simulink library "Feuchtesimulation_Lib"  (R2018b)
settings: Solver=VariableStepAuto  StartTime=0.0  StopTime=10.0  RelTol=1e-3
undefined symbols (not defined in the file or in its folder): A_Kat0, A_Mantel_Kat0, Ads_AusnutzungsFaktor, adsorptionsenthalpie, AIR_mw, beladungskennfeld, c_edelstahl, c_Isomatte, deltaH_verd, DiscIntNeverNeededParam, H2O_mw, Kat0_Anzahl_Zonen, Kond_AusnutzungsFaktor, Kond_KL_Faktor_, KondVerd_KLKF_mf_StSt_kgps, l_Kat0, m_Canning_Kat0, m_h2o_kat0_ads, m_h2o_kat0_kond, m_Isolierung_Kat0, m_zeolith_kat0_zone, m_zKat0, Mat_Kat0, mGas_imRohrabschnitt_kg, mZeo_UnterDerZeo0angenommenWird, p_dsat, R_sLuft, rate_k_verd, Rohr1, RTh_Brick_Iso_Kat0, RTh_Iso_Canning_Kat0, Sensor0, SensorIn, switch_TInit_Tstart_bei_true_sonst_TInitAusMessung, T_start, Tk0_1, ts, Verd_KF_Dampfdruck_StSt, Verd_KL_Faktor, waermekapazitaet_luft, waermekapazitaet_wasser_fluessig, waermekapazitaet_wasser_gasfoermig, WuezRohr_Dynamikfaktor
libraries: simulink x5, $bdroot x3
(part 1 of 2)
settings Model: Creator=QXS2633  LastModifiedBy=qt28407

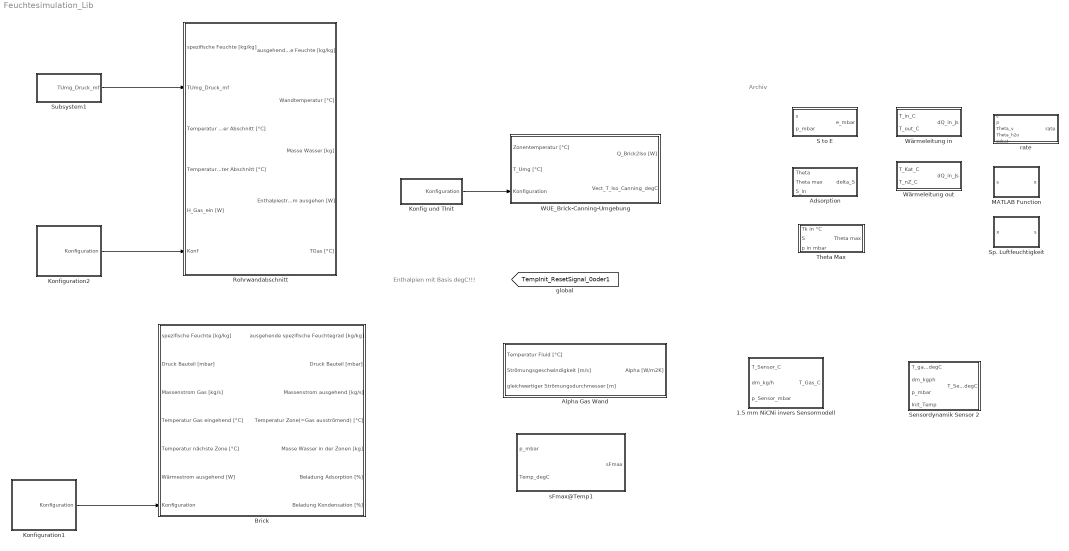
== system Feuchtesimulation_Lib ==
  note: Archiv
  note: Enthalpien mit Basis degC!!!
  1.5 mm NiCNi invers Sensormodell : Subsystem
  Adsorption : Subsystem
  Alpha Gas Wand : Subsystem
  Brick : Subsystem
  Konfig und TInit : Subsystem
  Konfiguration1 : Subsystem
  Konfiguration2 : Subsystem
  MATLAB Function : MATLAB Function  TreatAsAtomicUnit=on
  Rohrwandabschnitt : Subsystem
  S to E : Subsystem
  Sensordynamik Sensor 2 : Subsystem
  Sp. Luftfeuchtigkeit : MATLAB Function  TreatAsAtomicUnit=on
  Subsystem1 : Subsystem
  Theta Max : Subsystem
  WUE_Brick-Canning-Umgebung : Subsystem
  Wärmeleitung in : Subsystem
  Wärmeleitung out : Subsystem
  rate : Subsystem
  sFmax@Temp1 : MATLAB Function  TreatAsAtomicUnit=on
  tag scope: TempInit_ResetSignal_0oder1=global
  wires:
  Konfiguration1/1(Konfiguration) -> Brick/7(Konfiguration)
  Konfiguration2/1(Konfiguration) -> Rohrwandabschnitt/6(Konf)
  Subsystem1/1(TUmg_Druck_mf) -> Rohrwandabschnitt/2(TUmg_Druck_mf)
  Konfig und TInit/1(Konfiguration) -> WUE_Brick-Canning-Umgebung/3(Konfiguration)

== system Feuchtesimulation_Lib/1.5 mm NiCNi invers Sensormodell ==
  T_Sensor_C : Inport
  dm_kg/h : Inport  Port=2
  p_Sensor_mbar : Inport  Port=3
  dm_to_v : Subsystem
  erh. Sensordynamik : Subsystem
  T_Gas_C : Outport
  wires:
  dm_kg/h/1 -> dm_to_v/1(dm_kg/h)
  dm_to_v/1(v_m/s) -> erh. Sensordynamik/2(v_m/s)
  T_Sensor_C/1 -> dm_to_v/3(Tg_C), erh. Sensordynamik/1(T_in_c)
  p_Sensor_mbar/1 -> dm_to_v/2(p_mbar)
  erh. Sensordynamik/1(T_out_c) -> T_Gas_C/1

== system Feuchtesimulation_Lib/Adsorption ==
  Theta : Inport
  Theta max : Inport  Port=2
  S_in : Inport  Port=3
  Assertion : Assertion
  Constant : Constant
  Divide : Product  Inputs=*/
  Multiply : Product
  Sum : Sum  Inputs=+-|
  delta_S : Outport
  wires:
  Theta max/1 -> Assertion/1, Divide/2
  Theta/1 -> Divide/1
  Divide/1 -> Sum/2
  Constant/1 -> Sum/1
  Sum/1 -> Multiply/1
  Multiply/1 -> delta_S/1
  S_in/1 -> Multiply/2

== system Feuchtesimulation_Lib/Alpha Gas Wand ==
  Temperatur Fluid [°C] : Inport
  Strömungsgeschwindigkeit [m/s] : Inport  Port=2
  gleichwertiger Strömungsdurchmesser [m] : Inport  Port=3
  MATLAB Function : MATLAB Function  TreatAsAtomicUnit=on
  Alpha [W/m2K] : Outport
  wires:
  MATLAB Function/1(alpha) -> Alpha [W/m2K]/1
  Temperatur Fluid [°C]/1 -> MATLAB Function/1(tf)
  Strömungsgeschwindigkeit [m/s]/1 -> MATLAB Function/2(v)
  gleichwertiger Strömungsdurchmesser [m]/1 -> MATLAB Function/3(dgl)

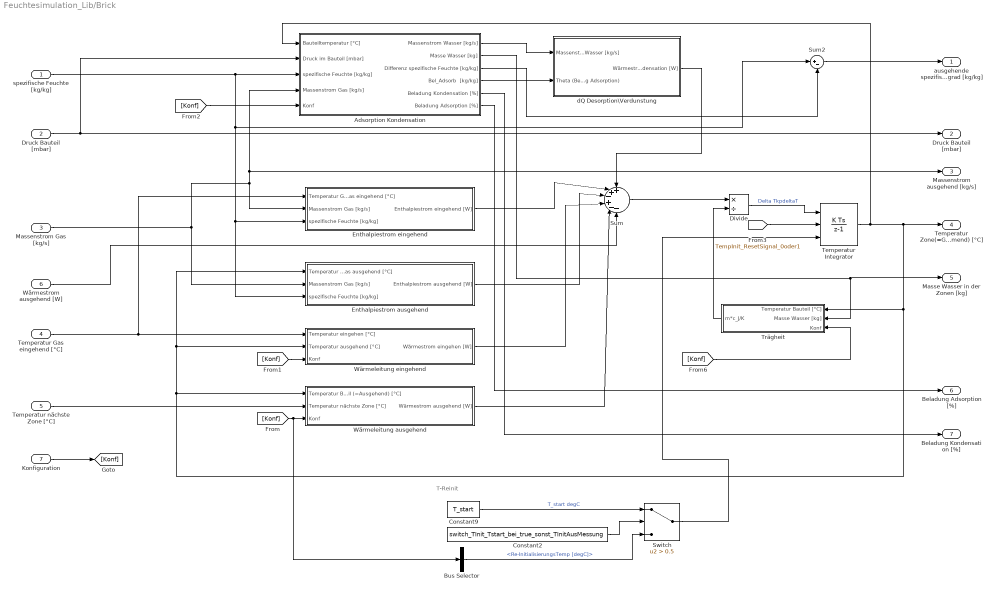
== system Feuchtesimulation_Lib/Brick ==
  note: T-Reinit
  spezifische Feuchte [kg/kg] : Inport
  Druck Bauteil [mbar] : Inport  Port=2
  "Massenstrom Gas [kg/s] " : Inport  Port=3
  Temperatur Gas eingehend [°C] : Inport  Port=4
  Temperatur nächste Zone [°C] : Inport  Port=5
  Wärmestrom ausgehend [W] : Inport  Port=6
  Konfiguration : Inport  Port=7
  Adsorption Kondensation : Subsystem
  Bus Selector : BusSelector  OutputSignals=Re-InitialisierungsTemp [degC]
  Constant2 : Constant  Value=switch_TInit_Tstart_bei_true_sonst_TInitAusMessung
  Constant9 : Constant  Value=T_start
  Divide : Product  Inputs=*/
  "Enthalpiestrom ausgehend " : Subsystem
  "Enthalpiestrom eingehend " : Subsystem
  Sum : Sum  Inputs=++-+--
  Sum2 : Sum  Inputs=|+-
  Switch : Switch  Criteria=u2 > Threshold  Threshold=0.5
  Temperatur Integrator : DiscreteIntegrator  ExternalReset=rising  InitialConditionSource=external  InitialCondition=Tk0_1  SampleTime=ts  ICPrevOutput=DiscIntNeverNeededParam  ICPrevScaledInput=DiscIntNeverNeededParam
  "Trägheit " : Subsystem
  "Wärmeleitung ausgehend " : Subsystem
  Wärmeleitung eingehend : Subsystem
  dQ Desorption\Verdunstung : Subsystem
  ausgehende spezifische Feuchtegrad [kg/kg] : Outport
  "Druck Bauteil [mbar] " : Outport  Port=2
  Massenstrom ausgehend [kg/s] : Outport  Port=3
  Temperatur Zone(=Gas ausströmend) [°C] : Outport  Port=4
  Masse Wasser in der Zonen [kg] : Outport  Port=5
  Beladung Adsorption [%] : Outport  Port=6
  Beladung Kondensation [%] : Outport  Port=7
  wires:
  Wärmeleitung eingehend/1(Wärmestrom eingehen [W]) -> Sum/4
  "Wärmeleitung ausgehend "/1(Wärmestrom ausgehend [W]) -> Sum/5
  "Enthalpiestrom ausgehend "/1(Enthalpiestrom ausgehend [W]) -> Sum/3
  Temperatur Gas eingehend [°C]/1 -> "Enthalpiestrom eingehend "/1(Temperatur Gas eingehend [°C]), Wärmeleitung eingehend/1(Temperatur eingehen [°C])
  Temperatur nächste Zone [°C]/1 -> "Wärmeleitung ausgehend "/2(Temperatur nächste Zone [°C])
  Divide/1 -> Temperatur Integrator/1  "Delta TkpdeltaT"
  "Enthalpiestrom eingehend "/1(Enthalpiestrom eingehend [W]) -> Sum/2
  spezifische Feuchte [kg/kg]/1 -> Sum2/1, "Enthalpiestrom ausgehend "/3(spezifische Feuchte [kg/kg]), "Enthalpiestrom eingehend "/3(spezifische Feuchte [kg/kg]), Adsorption Kondensation/3(spezifische Feuchte [kg/kg])
  Sum/1 -> Divide/1
  "Massenstrom Gas [kg/s] "/1 -> "Enthalpiestrom eingehend "/2(Massenstrom Gas [kg/s]), Adsorption Kondensation/4(Massenstrom Gas [kg/s]), Massenstrom ausgehend [kg/s]/1, "Enthalpiestrom ausgehend "/2(Massenstrom Gas [kg/s])
  Druck Bauteil [mbar]/1 -> Adsorption Kondensation/2(Druck im Bauteil [mbar]), "Druck Bauteil [mbar] "/1
  Adsorption Kondensation/1(Massenstrom Wasser [kg/s]) -> dQ Desorption\Verdunstung/1(Massenstrom Wasser [kg/s])
  dQ Desorption\Verdunstung/1(Wärmestrom Adsorption/Kondensation [W]) -> Sum/1
  Adsorption Kondensation/2(Masse Wasser [kg]) -> "Trägheit "/2(Masse Wasser [kg]), Masse Wasser in der Zonen [kg]/1
  Temperatur Integrator/1 -> Adsorption Kondensation/1(Bauteiltemperatur [°C]), Temperatur Zone(=Gas ausströmend) [°C]/1, "Enthalpiestrom ausgehend "/1(Temperatur Gas ausgehend [°C]), Wärmeleitung eingehend/2(Temperatur ausgehend [°C]), "Wärmeleitung ausgehend "/1(Temperatur Bauteil (=Ausgehend) [°C]), "Trägheit "/1(Temperatur Bauteil [°C])
  "Trägheit "/1(m*c_J/K) -> Divide/2
  Konfiguration/1 -> [Konf]
  [Konf] -> Bus Selector/1, "Wärmeleitung ausgehend "/3(Konf)
  [Konf] -> Wärmeleitung eingehend/3(Konf)
  [Konf] -> "Trägheit "/3(Konf)
  Sum2/1 -> ausgehende spezifische Feuchtegrad [kg/kg]/1
  Adsorption Kondensation/3(Differenz spezifische Feuchte [kg/kg]) -> Sum2/2
  [Konf] -> Adsorption Kondensation/5(Konf)
  Adsorption Kondensation/5(Beladung Kondensation [%]) -> Beladung Kondensation [%]/1
  Wärmestrom ausgehend [W]/1 -> Sum/6
  Adsorption Kondensation/6(Beladung Adsorption [%]) -> Beladung Adsorption [%]/1
  Adsorption Kondensation/4(Bel_Adsorb  [kg/kg]) -> dQ Desorption\Verdunstung/2(Theta (Beladung Adsorption))
  [TempInit_ResetSignal_0oder1] -> Temperatur Integrator/2
  Constant9/1 -> Switch/1  "T_start degC"
  Constant2/1 -> Switch/2
  Bus Selector/1 -> Switch/3  "<Re-InitialisierungsTemp [degC]>"
  Switch/1 -> Temperatur Integrator/3

== system Feuchtesimulation_Lib/Konfig und TInit ==
  Bus Creator : BusCreator  Inputs=7
  Constant : Constant  Value=RTh_Brick_Iso_Kat0
  Constant1 : Constant  Value=RTh_Iso_Canning_Kat0
  Constant2 : Constant  Value=m_Isolierung_Kat0
  Constant3 : Constant  Value=m_Canning_Kat0
  Constant4 : Constant  Value=A_Mantel_Kat0
  Constant5 : Constant  Value=Kat0_Anzahl_Zonen
  From Workspace : FromWorkspace  VariableName=simin  SampleTime=0
  Konfiguration : Outport
  wires:
  Bus Creator/1 -> Konfiguration/1
  Constant/1 -> Bus Creator/1  "RTh_Brick_Iso [K/W]"
  Constant1/1 -> Bus Creator/2  "RTh_Iso_Canning [K/W]"
  Constant3/1 -> Bus Creator/4  "m_Canning [kg]"
  Constant4/1 -> Bus Creator/5  "A_Mantel [m2]"
  Constant5/1 -> Bus Creator/6  "Anzahl_Zonen [-]"
  Constant2/1 -> Bus Creator/3  "m_Isolierung [kg]"
  From Workspace/1 -> Bus Creator/7  "Re-InitialisierungsTemp [degC]"

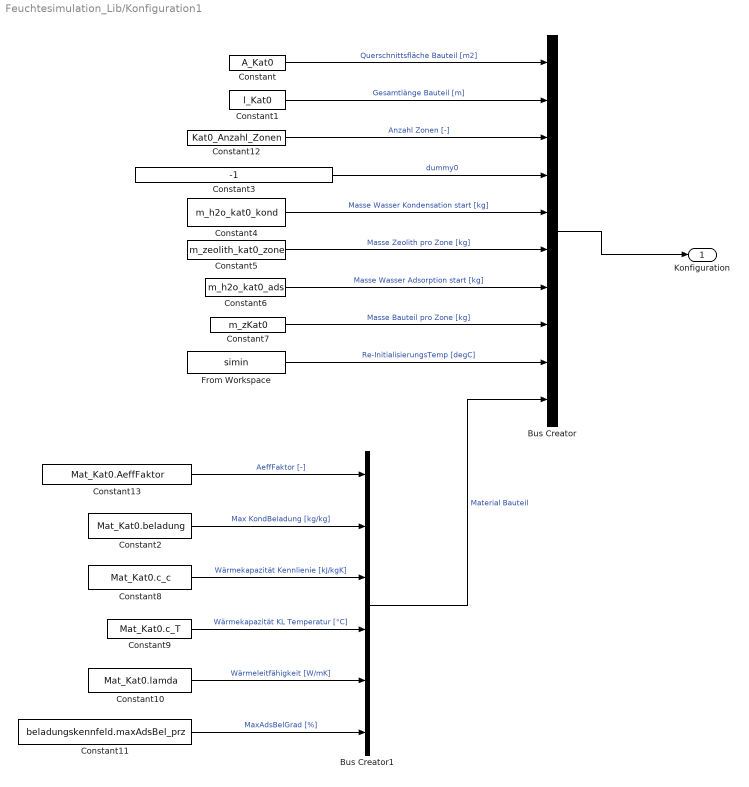
== system Feuchtesimulation_Lib/Konfiguration1 ==
  Bus Creator : BusCreator  Inputs=10
  Bus Creator1 : BusCreator  Inputs=6
  Constant : Constant  Value=A_Kat0
  Constant1 : Constant  Value=l_Kat0
  Constant10 : Constant  Value=Mat_Kat0.lamda
  Constant11 : Constant  Value=beladungskennfeld.maxAdsBel_prz
  Constant12 : Constant  Value=Kat0_Anzahl_Zonen
  Constant13 : Constant  Value=Mat_Kat0.AeffFaktor
  Constant2 : Constant  Value=Mat_Kat0.beladung
  Constant3 : Constant  Value=-1
  Constant4 : Constant  Value=m_h2o_kat0_kond
  Constant5 : Constant  Value=m_zeolith_kat0_zone
  Constant6 : Constant  Value=m_h2o_kat0_ads
  Constant7 : Constant  Value=m_zKat0
  Constant8 : Constant  Value=Mat_Kat0.c_c
  Constant9 : Constant  Value=Mat_Kat0.c_T
  From Workspace : FromWorkspace  VariableName=simin  SampleTime=0
  Konfiguration : Outport
  wires:
  Bus Creator/1 -> Konfiguration/1
  Constant/1 -> Bus Creator/1  "Querschnittsfläche Bauteil [m2]"
  Constant1/1 -> Bus Creator/2  "Gesamtlänge Bauteil [m]"
  Constant4/1 -> Bus Creator/5  "Masse Wasser Kondensation start [kg]"
  Constant5/1 -> Bus Creator/6  "Masse Zeolith pro Zone [kg]"
  Constant6/1 -> Bus Creator/7  "Masse Wasser Adsorption start [kg]"
  Constant7/1 -> Bus Creator/8  "Masse Bauteil pro Zone [kg]"
  Bus Creator1/1 -> Bus Creator/10  "Material Bauteil"
  Constant2/1 -> Bus Creator1/2  "Max KondBeladung [kg/kg]"
  Constant8/1 -> Bus Creator1/3  "Wärmekapazität Kennlienie [kJ/kgK]"
  Constant9/1 -> Bus Creator1/4  "Wärmekapazität KL Temperatur [°C]"
  Constant10/1 -> Bus Creator1/5  "Wärmeleitfähigkeit [W/mK]"
  Constant12/1 -> Bus Creator/3  "Anzahl Zonen [-]"
  Constant13/1 -> Bus Creator1/1  "AeffFaktor [-]"
  Constant11/1 -> Bus Creator1/6  "MaxAdsBelGrad [%]"
  From Workspace/1 -> Bus Creator/9  "Re-InitialisierungsTemp [degC]"
  Constant3/1 -> Bus Creator/4  "dummy0"

== system Feuchtesimulation_Lib/Konfiguration2 ==
  Bus Creator : BusCreator  Inputs=13
  Constant : Constant  Value=Rohr1.Mantelflaeche_innen
  Constant1 : Constant  Value=Rohr1.Mantelflaeche_aussen
  Constant12 : Constant  Value=Rohr1.Laenge_Abschnitt
  Constant15 : Constant  Value=Rohr1.Waermeleitquerschnitt
  Constant2 : Constant  Value=Rohr1.StroemungsdurchmesserEff
  Constant3 : Constant  Value=Rohr1.thermWidIso
  Constant4 : Constant  Value=Rohr1.Masse_Wasser_start
  Constant5 : Constant  Value=Rohr1.LambdaRohr
  Constant6 : Constant  Value=Rohr1.MasseRohr
  Constant7 : Constant  Value=Rohr1.Kondensationskoeffizient
  Constant8 : Constant  Value=Rohr1.Waermekapazitaet
  Constant9 : Constant  Value=Rohr1.thermWidRohr
  From Workspace : FromWorkspace  VariableName=simin  SampleTime=0
  Konfiguration : Outport
  wires:
  Bus Creator/1 -> Konfiguration/1
  Constant/1 -> Bus Creator/1  "Mantelfläche innen [m2]"
  Constant1/1 -> Bus Creator/2  "Mantelfläche außen [m2]"
  Constant4/1 -> Bus Creator/5  "Masse Wasser start [kg]"
  Constant12/1 -> Bus Creator/3  "Länge RohrSegment [m]"
  Constant15/1 -> Bus Creator/11  "Wärmeleitquerschnitt Rohr [m2]"
  Constant2/1 -> Bus Creator/7  "gleichwertiger Strömungsdurchmesser [m]"
  Constant5/1 -> Bus Creator/8  "Wärmeleitfähigkeit [W/mK]"
  Constant6/1 -> Bus Creator/9  "Masse Rohr [kg]"
  Constant8/1 -> Bus Creator/10  "Wärmekapazität Rohr [J/kgK]"
  Constant7/1 -> Bus Creator/12  "Kondensationskoeffizient"
  From Workspace/1 -> Bus Creator/13  "Re-InitialisierungsTemp [degC]"
  Constant3/1 -> Bus Creator/4  "r_thermWidIso_m2K/W"
  Constant9/1 -> Bus Creator/6  "r_thermWidRohr_m2K/W"

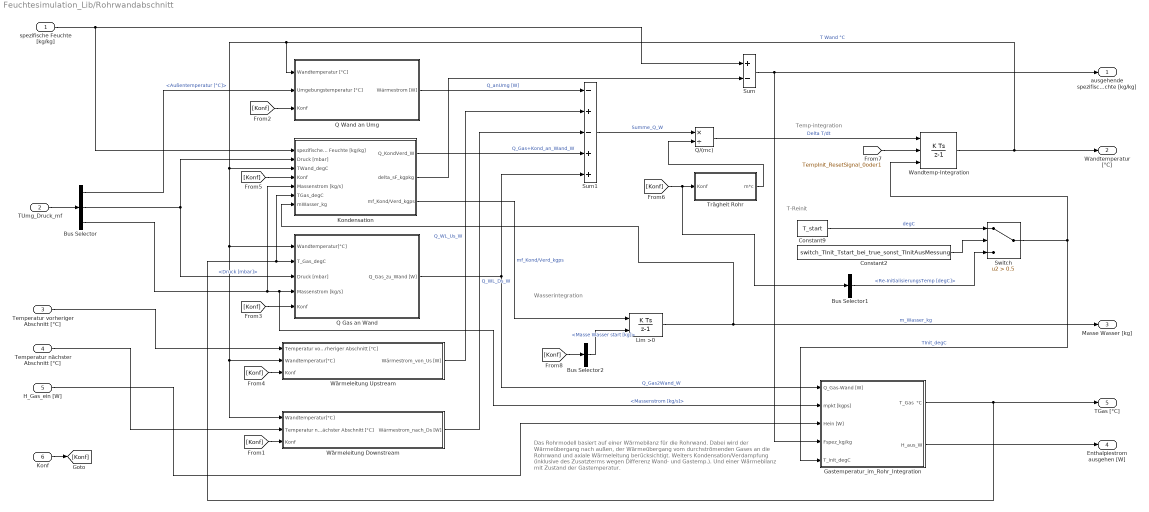
== system Feuchtesimulation_Lib/Rohrwandabschnitt ==
  note: Wasserintegration
  note: Das Rohrmodell basiert auf einer Wärmebilanz für die Rohrwand.
      | Dabei wird der Wärmeübergang nach außen, der Wärmeübergang
      | vom durchströmenden Gases an die Rohrwand und axiale
      | Wärmeleitung berücksichtigt.
      | Weiters Kondensation/Verdampfung (inklusive des Zusatzterms
      | wegen Differenz Wand- und Gastemp.).
      | Und einer Wärmebilanz mit Zustand der Gastemperatur.
  note: T-Reinit
  note: Temp-integration
  spezifische Feuchte [kg/kg] : Inport
  TUmg_Druck_mf : Inport  Port=2
  Temperatur vorheriger Abschnitt [°C] : Inport  Port=3
  Temperatur nächster Abschnitt [°C] : Inport  Port=4
  H_Gas_ein [W] : Inport  Port=5
  Konf : Inport  Port=6
  Bus Selector : BusSelector  OutputSignals=Außentemperatur [°C],Druck [mbar],Massenstrom [kg/s]
  Bus Selector1 : BusSelector  OutputSignals=Re-InitialisierungsTemp [degC]
  Bus Selector2 : BusSelector  OutputSignals=Masse Wasser start [kg]
  Constant2 : Constant  Value=switch_TInit_Tstart_bei_true_sonst_TInitAusMessung
  Constant9 : Constant  Value=T_start
  Gastemperatur_im_Rohr_Integration : Subsystem
  Kondensation : Subsystem
  Lim >0 : DiscreteIntegrator  InitialConditionSource=external  SampleTime=-1  LimitOutput=on  LowerSaturationLimit=0  ICPrevOutput=DiscIntNeverNeededParam  ICPrevScaledInput=DiscIntNeverNeededParam
  Q Gas an Wand : Subsystem
  Q Wand an Umg : Subsystem
  Q/(mc) : Product  Inputs=*/
  Sum : Sum  Inputs=+-
  Sum1 : Sum  Inputs=-+-++
  Switch : Switch  Criteria=u2 > Threshold  Threshold=0.5
  Trägheit Rohr : Subsystem
  Wandtemp-Integration : DiscreteIntegrator  ExternalReset=rising  InitialConditionSource=external  SampleTime=-1  ICPrevOutput=DiscIntNeverNeededParam  ICPrevScaledInput=DiscIntNeverNeededParam
  Wärmeleitung Downstream : Subsystem
  Wärmeleitung Upstream : Subsystem
  ausgehende spezifische Feuchte [kg/kg] : Outport
  Wandtemperatur [°C] : Outport  Port=2
  Masse Wasser [kg] : Outport  Port=3
  Enthalpiestrom ausgehen [W] : Outport  Port=4
  TGas [°C] : Outport  Port=5
  wires:
  Bus Selector/3 -> Q Gas an Wand/4(Massenstrom [kg/s]), Gastemperatur_im_Rohr_Integration/2(mpkt [kgps]), Kondensation/5(Massenstrom [kg/s])  "<Massenstrom [kg/s]>"
  Sum1/1 -> Q/(mc)/1  "Summe_Q_W"
  Q/(mc)/1 -> Wandtemp-Integration/1  "Delta T/dt"
  Trägheit Rohr/1(m*c) -> Q/(mc)/2
  Wandtemp-Integration/1 -> Wärmeleitung Downstream/1(Wandtemperatur[°C]), Wärmeleitung Upstream/2(Wandtemperatur[°C]), Q Gas an Wand/1(Wandtemperatur[°C]), Kondensation/3(TWand_degC), Q Wand an Umg/1(Wandtemperatur [°C]), Wandtemperatur [°C]/1  "T Wand °C"
  Bus Selector/2 -> Kondensation/2(Druck [mbar]), Q Gas an Wand/3(Druck [mbar])  "<Druck [mbar]>"
  Lim >0/1 -> Masse Wasser [kg]/1, Kondensation/7(mWasser_kg)  "m_Wasser_kg"
  H_Gas_ein [W]/1 -> Gastemperatur_im_Rohr_Integration/3(Hein [W])
  spezifische Feuchte [kg/kg]/1 -> Sum/1, Kondensation/1(spezifische Feuchte [kg/kg])
  Konf/1 -> [Konf]
  [Konf] -> Wärmeleitung Downstream/3(Konf)
  [Konf] -> Q Wand an Umg/3(Konf)
  [Konf] -> Q Gas an Wand/5(Konf)
  [Konf] -> Wärmeleitung Upstream/3(Konf)
  Q Wand an Umg/1(Wärmestrom [W]) -> Sum1/1  "Q_anUmg [W]"
  Q Gas an Wand/1(Q_Gas_zu_Wand [W]) -> Sum1/5, Gastemperatur_im_Rohr_Integration/1(Q_Gas-Wand [W])  "Q_Gas2Wand_W"
  [Konf] -> Kondensation/4(Konf)
  [Konf] -> Bus Selector1/1, Trägheit Rohr/1(Konf)
  Temperatur nächster Abschnitt [°C]/1 -> Wärmeleitung Downstream/2(Temperatur nächster Abschnitt [°C])
  TUmg_Druck_mf/1 -> Bus Selector/1
  Bus Selector/1 -> Q Wand an Umg/2(Umgebungstemperatur [°C])  "<Außentemperatur [°C]>"
  Sum/1 -> Gastemperatur_im_Rohr_Integration/4(Fspez_kg/kg), ausgehende spezifische Feuchte [kg/kg]/1
  Kondensation/2(delta_sF_kgpkg) -> Sum/2
  Wärmeleitung Downstream/1(Wärmestrom_nach_Ds [W]) -> Sum1/3  "Q_WL_Ds_W"
  Wärmeleitung Upstream/1(Wärmestrom_von_Us [W]) -> Sum1/2  "Q_WL_Us_W"
  Temperatur vorheriger Abschnitt [°C]/1 -> Wärmeleitung Upstream/1(Temperatur vorheriger Abschnitt [°C])
  Gastemperatur_im_Rohr_Integration/1(T_Gas  °C) -> TGas [°C]/1, Q Gas an Wand/2(T_Gas_degC), Kondensation/6(TGas_degC)
  Constant2/1 -> Switch/2
  Constant9/1 -> Switch/1  "degC"
  Switch/1 -> Wandtemp-Integration/3, Gastemperatur_im_Rohr_Integration/5(T_init_degC)  "TInit_degC"
  [TempInit_ResetSignal_0oder1] -> Wandtemp-Integration/2
  Bus Selector1/1 -> Switch/3  "<Re-InitialisierungsTemp [degC]>"
  [Konf] -> Bus Selector2/1
  Gastemperatur_im_Rohr_Integration/2(H_aus_W) -> Enthalpiestrom ausgehen [W]/1
  Bus Selector2/1 -> Lim >0/2  "<Masse Wasser start [kg]>"
  Kondensation/3(mf_Kond/Verd_kgps) -> Lim >0/1  "mf_Kond/Verd_kgps"
  Kondensation/1(Q_KondVerd_W) -> Sum1/4  "Q_Gas+Kond_an_Wand_W"

== system Feuchtesimulation_Lib/S to E ==
  s : Inport
  p_mbar : Inport  Port=2
  Constant : Constant  Value=H2O_mw/AIR_mw
  Divide : Product  Inputs=*/
  Multiply : Product
  Multiply1 : Product
  Sum : Sum  Inputs=++-
  e_mbar : Outport
  wires:
  s/1 -> Multiply1/1, Sum/1, Multiply/1
  p_mbar/1 -> Multiply/2
  Multiply/1 -> Divide/1
  Multiply1/1 -> Sum/3
  Constant/1 -> Sum/2, Multiply1/2
  Sum/1 -> Divide/2
  Divide/1 -> e_mbar/1

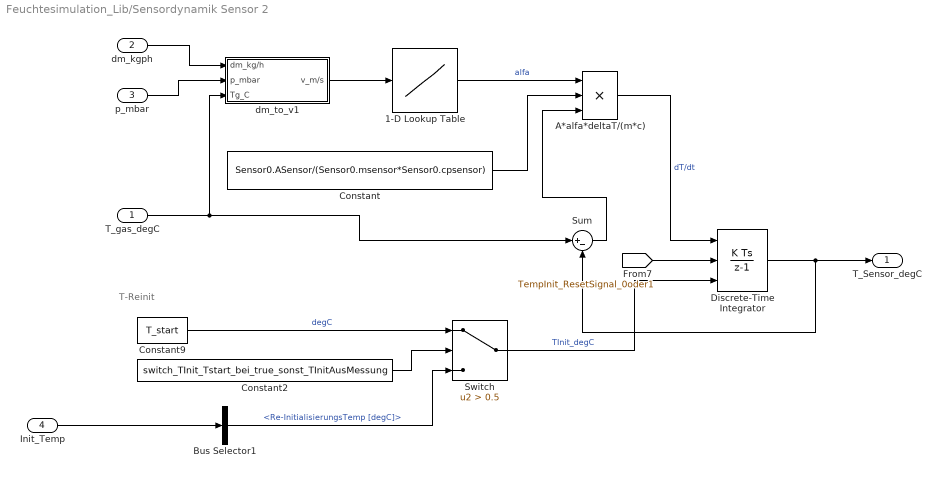
== system Feuchtesimulation_Lib/Sensordynamik Sensor 2 ==
  note: T-Reinit
  T_gas_degC : Inport
  dm_kgph : Inport  Port=2
  p_mbar : Inport  Port=3
  Init_Temp : Inport  Port=4
  1-D Lookup Table : Lookup_n-D  NumberOfTableDimensions=1  BreakpointsForDimension1=Sensor0.wuez_v  Table=Sensor0.wuez_alpha  InternalRulePriority=Speed  RndMeth=Simplest  InputSameDT=on
  A*alfa*deltaT/(m*c) : Product  Inputs=3
  Bus Selector1 : BusSelector  OutputSignals=Re-InitialisierungsTemp [degC]
  Constant : Constant  Value=Sensor0.ASensor/(Sensor0.msensor*Sensor0.cpsensor)
  Constant2 : Constant  Value=switch_TInit_Tstart_bei_true_sonst_TInitAusMessung
  Constant9 : Constant  Value=T_start
  Discrete-Time Integrator : DiscreteIntegrator  ExternalReset=rising  InitialConditionSource=external  SampleTime=ts  UpperSaturationLimit=500  LowerSaturationLimit=0  ICPrevOutput=DiscIntNeverNeededParam  ICPrevScaledInput=DiscIntNeverNeededParam
  Sum : Sum  Inputs=|+-
  Switch : Switch  Criteria=u2 > Threshold  Threshold=0.5
  dm_to_v1 : Subsystem
  T_Sensor_degC : Outport
  wires:
  Constant/1 -> A*alfa*deltaT/(m*c)/2
  Sum/1 -> A*alfa*deltaT/(m*c)/3
  1-D Lookup Table/1 -> A*alfa*deltaT/(m*c)/1  "alfa"
  dm_to_v1/1(v_m/s) -> 1-D Lookup Table/1
  A*alfa*deltaT/(m*c)/1 -> Discrete-Time Integrator/1  "dT/dt"
  Discrete-Time Integrator/1 -> T_Sensor_degC/1, Sum/2
  T_gas_degC/1 -> dm_to_v1/3(Tg_C), Sum/1
  p_mbar/1 -> dm_to_v1/2(p_mbar)
  dm_kgph/1 -> dm_to_v1/1(dm_kg/h)
  Constant9/1 -> Switch/1  "degC"
  Constant2/1 -> Switch/2
  Init_Temp/1 -> Bus Selector1/1
  Bus Selector1/1 -> Switch/3  "<Re-InitialisierungsTemp [degC]>"
  [TempInit_ResetSignal_0oder1] -> Discrete-Time Integrator/2
  Switch/1 -> Discrete-Time Integrator/3  "TInit_degC"

== system Feuchtesimulation_Lib/Subsystem1 ==
  Bus Creator : BusCreator  Inputs=3
  From Workspace : FromWorkspace  VariableName=simin  SampleTime=0
  From Workspace1 : FromWorkspace  VariableName=simin  SampleTime=0
  From Workspace2 : FromWorkspace  VariableName=simin  SampleTime=0
  TUmg_Druck_mf : Outport
  wires:
  From Workspace/1 -> Bus Creator/1  "Außentemperatur [°C]"
  From Workspace2/1 -> Bus Creator/3  "Massenstrom [kg/s]"
  From Workspace1/1 -> Bus Creator/2  "Druck [mbar]"
  Bus Creator/1 -> TUmg_Druck_mf/1

== system Feuchtesimulation_Lib/Theta Max ==
  Tk in °C : Inport
  S : Inport  Port=2
  p in mbar : Inport  Port=3
  % to 1 : Gain  Gain=0.01
  2-D Lookup Table : Lookup_n-D  BreakpointsForDimension1=beladungskennfeld.T  BreakpointsForDimension2=beladungskennfeld.e  Table=beladungskennfeld.table  InternalRulePriority=Speed  RndMeth=Simplest  InputSameDT=on
  S to E : $bdroot/S to E  SystemSampleTime=-1
  mbar to pa : Gain  Gain=100
  Theta max : Outport
  wires:
  S to E/1 -> mbar to pa/1
  Tk in °C/1 -> 2-D Lookup Table/1
  p in mbar/1 -> S to E/2
  S/1 -> S to E/1
  2-D Lookup Table/1 -> % to 1/1
  % to 1/1 -> Theta max/1
  mbar to pa/1 -> 2-D Lookup Table/2

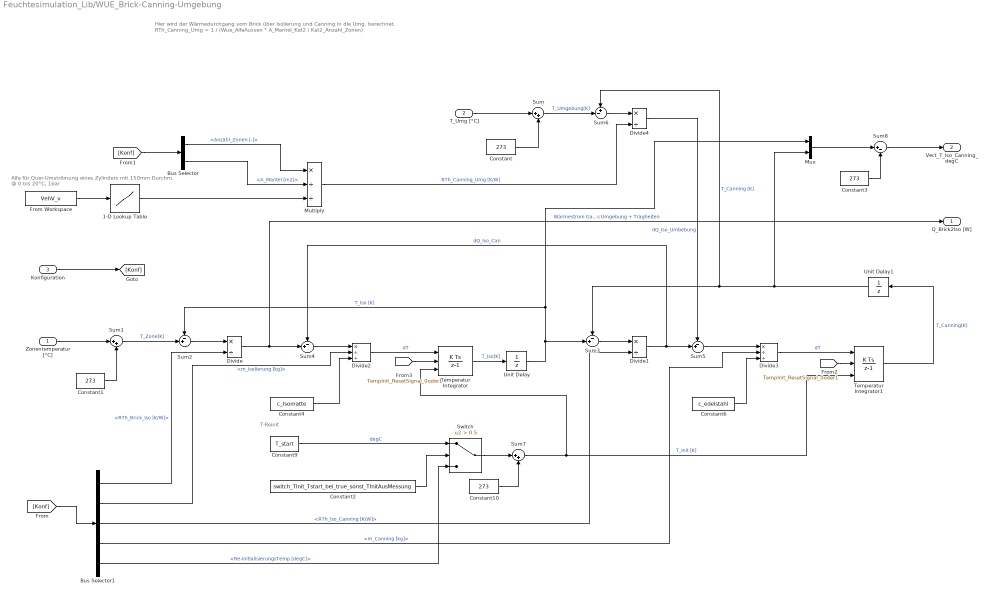
== system Feuchtesimulation_Lib/WUE_Brick-Canning-Umgebung ==
  note: T-Reinit
  note: Hier wird der Wärmedurchgang vom Brick über Isolierung und Canning in die Umg.
      | berechnet.
      |
      | RTh_Canning_Umg = 1 / (Wue_AlfaAussen * A_Mantel_Kat2 / Kat2_Anzahl_Zonen)
  note: Alfa für Quer-Umströmung eines Zylinders mit 150mm Durchm.
      | @ 0 bis 20°C, 1bar
  Zonentemperatur [°C] : Inport
  T_Umg [°C] : Inport  Port=2
  Konfiguration : Inport  Port=3
  1-D Lookup Table : Lookup_n-D  NumberOfTableDimensions=1  BreakpointsForDimension1=[0, 10, 20, 50, 100, 200, 300]  Table=[8, 18, 32, 66, 116, 200, 280]  InternalRulePriority=Speed  RndMeth=Simplest  InputSameDT=on
  Bus Selector : BusSelector  OutputSignals=Anzahl_Zonen [-],A_Mantel [m2]
  Bus Selector1 : BusSelector  OutputSignals=RTh_Brick_Iso [K/W],m_Isolierung [kg],RTh_Iso_Canning [K/W],m_Canning [kg],Re-InitialisierungsTemp [degC]
  Constant{,1,3,10} (4 alike) : Constant  Value=273
  Constant2 : Constant  Value=switch_TInit_Tstart_bei_true_sonst_TInitAusMessung
  Constant4 : Constant  Value=c_Isomatte
  Constant6 : Constant  Value=c_edelstahl
  Constant9 : Constant  Value=T_start
  Divide : Product  Inputs=*/
  Divide1 : Product  Inputs=*/
  Divide2 : Product  Inputs=*//
  Divide3 : Product  Inputs=*//
  Divide4 : Product  Inputs=*/
  From Workspace : FromWorkspace  VariableName=VehV_v  SampleTime=0
  Multiply : Product  Inputs=*//
  Mux : Mux  Inputs=2
  Sum : Sum  Inputs=|++
  Sum1 : Sum  Inputs=|++
  Sum{2..5} (4 alike) : Sum  Inputs=-+|
  Sum6 : Sum  Inputs=+-|
  Sum7 : Sum  Inputs=|++
  Sum8 : Sum  Inputs=|+-
  Switch : Switch  Criteria=u2 > Threshold  Threshold=0.5
  Temperatur Integrator : DiscreteIntegrator  ExternalReset=rising  InitialConditionSource=external  InitialCondition=Tk0_1  SampleTime=ts  ICPrevOutput=DiscIntNeverNeededParam  ICPrevScaledInput=DiscIntNeverNeededParam
  Temperatur Integrator1 : DiscreteIntegrator  ExternalReset=rising  InitialConditionSource=external  InitialCondition=Tk0_1  SampleTime=ts  ICPrevOutput=DiscIntNeverNeededParam  ICPrevScaledInput=DiscIntNeverNeededParam
  Unit Delay : UnitDelay  InitialCondition=T_start+273  SampleTime=-1
  Unit Delay1 : UnitDelay  InitialCondition=T_start+273  SampleTime=-1
  Q_Brick2Iso [W] : Outport
  Vect_T_Iso_Canning_degC : Outport  Port=2
  wires:
  Divide/1 -> Q_Brick2Iso [W]/1, Sum4/2  "Wärmestrom Gas Umgebung + Trägheiten"
  Sum/1 -> Sum6/2  "T_Umgebung[K]"
  Constant/1 -> Sum/2
  T_Umg [°C]/1 -> Sum/1
  Zonentemperatur [°C]/1 -> Sum1/1
  Constant1/1 -> Sum1/2
  Sum1/1 -> Sum2/2  "T_Zone[K]"
  Unit Delay/1 -> Sum3/2, Mux/1, Sum2/1  "T_Iso [K]"
  Constant4/1 -> Divide2/3
  Temperatur Integrator/1 -> Unit Delay/1  "T_Iso[K]"
  Sum2/1 -> Divide/1
  Divide2/1 -> Temperatur Integrator/1  "dT"
  Divide3/1 -> Temperatur Integrator1/1  "dT"
  Sum3/1 -> Divide1/1
  Divide1/1 -> Sum4/1, Sum5/2  "dQ_Iso_Can"
  Constant6/1 -> Divide3/3
  Temperatur Integrator1/1 -> Unit Delay1/1  "T_Canning[K]"
  Unit Delay1/1 -> Mux/2, Sum3/1, Sum6/1  "T_Canning [K]"
  Sum4/1 -> Divide2/1
  Sum5/1 -> Divide3/1
  Multiply/1 -> Divide4/2  "RTh_Canning_Umg [K/W]"
  Divide4/1 -> Sum5/1  "dQ_Iso_Umbebung"
  Sum6/1 -> Divide4/1
  Konfiguration/1 -> [Konf]
  [Konf] -> Bus Selector1/1
  1-D Lookup Table/1 -> Multiply/3
  [Konf] -> Bus Selector/1
  Bus Selector/1 -> Multiply/1  "<Anzahl_Zonen [-]>"
  Bus Selector/2 -> Multiply/2  "<A_Mantel [m2]>"
  Bus Selector1/1 -> Divide/2  "<RTh_Brick_Iso [K/W]>"
  Bus Selector1/3 -> Divide1/2  "<RTh_Iso_Canning [K/W]>"
  Bus Selector1/2 -> Divide2/2  "<m_Isolierung [kg]>"
  Bus Selector1/4 -> Divide3/2  "<m_Canning [kg]>"
  [TempInit_ResetSignal_0oder1] -> Temperatur Integrator1/2
  [TempInit_ResetSignal_0oder1] -> Temperatur Integrator/2
  Constant9/1 -> Switch/1  "degC"
  From Workspace/1 -> 1-D Lookup Table/1
  Constant2/1 -> Switch/2
  Bus Selector1/5 -> Switch/3  "<Re-InitialisierungsTemp [degC]>"
  Constant10/1 -> Sum7/2
  Switch/1 -> Sum7/1
  Sum7/1 -> Temperatur Integrator/3, Temperatur Integrator1/3  "T_Init [K]"
  Constant3/1 -> Sum8/2
  Mux/1 -> Sum8/1
  Sum8/1 -> Vect_T_Iso_Canning_degC/1

== system Feuchtesimulation_Lib/Wärmeleitung in ==
  T_in_C : Inport
  T_out_C : Inport  Port=2
  A*lam/l_Js/K : Constant
  Multiply : Product
  Sum : Sum  Inputs=|+-
  dQ_in_Js : Outport
  wires:
  T_out_C/1 -> Sum/2
  T_in_C/1 -> Sum/1
  Sum/1 -> Multiply/2
  Multiply/1 -> dQ_in_Js/1
  A*lam/l_Js/K/1 -> Multiply/1

== system Feuchtesimulation_Lib/Wärmeleitung out ==
  T_Kat_C : Inport
  T_nZ_C : Inport  Port=2
  A*lam/l_Js/K : Constant
  Multiply : Product
  Sum : Sum  Inputs=|-+
  dQ_in_Js : Outport
  wires:
  T_nZ_C/1 -> Sum/2
  T_Kat_C/1 -> Sum/1
  Sum/1 -> Multiply/2
  Multiply/1 -> dQ_in_Js/1
  A*lam/l_Js/K/1 -> Multiply/1

== system Feuchtesimulation_Lib/rate ==
  s : Inport
  p : Inport  Port=2
  Theta_v : Inport  Port=3
  Theta_h2o : Inport  Port=4
  pdsat : Inport  Port=5
  Constant : Constant  Value=rate_k_verd
  Multiply : Product
  Multiply1 : Product
  Multiply2 : Product
  Sum : Sum  Inputs=+-
  s to e : Subsystem
  rate : Outport
  wires:
  s/1 -> s to e/1(s)
  p/1 -> s to e/2(p)
  Constant/1 -> Multiply/2
  Theta_v/1 -> Multiply1/2
  s to e/1(e) -> Multiply1/1
  Theta_h2o/1 -> Multiply2/2
  pdsat/1 -> Multiply2/1
  Multiply1/1 -> Sum/1
  Multiply2/1 -> Sum/2
  Sum/1 -> Multiply/1
  Multiply/1 -> rate/1

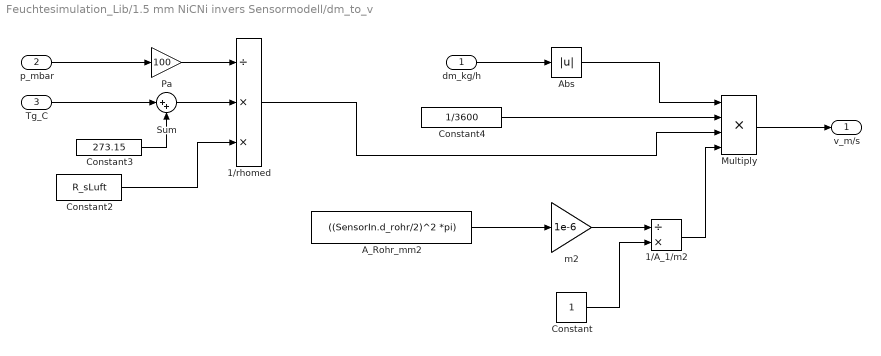
== system Feuchtesimulation_Lib/1.5 mm NiCNi invers Sensormodell/dm_to_v ==
  dm_kg/h : Inport
  p_mbar : Inport  Port=2
  Tg_C : Inport  Port=3
  1/A_1/m2 : Product  Inputs=/*
  1/rhomed : Product  Inputs=/**
  A_Rohr_mm2 : Constant  Value=((SensorIn.d_rohr/2)^2 *pi)
  Abs : Abs
  Constant : Constant
  Constant2 : Constant  Value=R_sLuft
  Constant3 : Constant  Value=273.15
  Constant4 : Constant  Value=1/3600
  Multiply : Product  Inputs=4
  Pa : Gain  Gain=100
  Sum : Sum  Inputs=|++
  m2 : Gain  Gain=1e-6
  v_m/s : Outport
  wires:
  dm_kg/h/1 -> Abs/1
  Constant4/1 -> Multiply/2
  1/rhomed/1 -> Multiply/3
  A_Rohr_mm2/1 -> m2/1
  m2/1 -> 1/A_1/m2/1
  Constant/1 -> 1/A_1/m2/2
  1/A_1/m2/1 -> Multiply/4
  Multiply/1 -> v_m/s/1
  Constant2/1 -> 1/rhomed/3
  Sum/1 -> 1/rhomed/2
  Tg_C/1 -> Sum/1
  Constant3/1 -> Sum/2
  p_mbar/1 -> Pa/1
  Pa/1 -> 1/rhomed/1
  Abs/1 -> Multiply/1

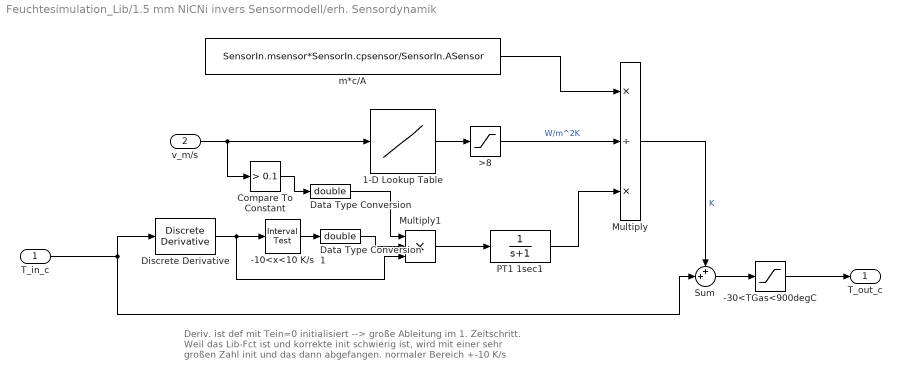
== system Feuchtesimulation_Lib/1.5 mm NiCNi invers Sensormodell/erh. Sensordynamik ==
  note: Deriv. ist def mit Tein=0 initialisiert --> große Ableitung im 1. Zeitschritt.
      | Weil das Lib-Fct ist und korrekte init schwierig ist, wird mit einer sehr
      | großen Zahl init und das dann abgefangen.
      |
      | normaler Bereich +-10 K/s
  T_in_c : Inport
  v_m/s : Inport  Port=2
  -10<x<10 K/s : simulink/Logic and Bit Operations/Interval Test  IntervalClosedRight=on  uplimit=10  IntervalClosedLeft=on  lowlimit=-10  OutDataTypeStr=uint8
  -30<TGas<900degC : Saturate  UpperLimit=900  LowerLimit=-30
  1-D Lookup Table : Lookup_n-D  NumberOfTableDimensions=1  BreakpointsForDimension1=SensorIn.wuez_v  IndexSearchMethod=Linear search  BeginIndexSearchUsingPreviousIndexResult=on  Table=SensorIn.wuez_alpha  ExtrapMethod=Clip  InternalRulePriority=Speed  RndMeth=Simplest  InputSameDT=on
  >8 : Saturate  UpperLimit=9e5  LowerLimit=8
  Compare To Constant : simulink/Logic and Bit Operations/Compare To Constant  relop=>  const=0.1  OutDataTypeStr=uint8
  Data Type Conversion : DataTypeConversion  OutDataTypeStr=double
  Data Type Conversion1 : DataTypeConversion  OutDataTypeStr=double
  Discrete Derivative : simulink/Discrete/Discrete Derivative  gainval=1.0  ICPrevScaledInput=99999  OutMin=[]  OutMax=[]  OutDataType=fixdt(1, 16)  OutScaling=2^-10  DoSatur=off
  Multiply : Product  Inputs=*/*
  Multiply1 : Product  Inputs=3
  PT1 1sec1 : TransferFcn  Denominator=[1 1]
  Sum : Sum  Inputs=++|
  m*c/A : Constant  Value=SensorIn.msensor*SensorIn.cpsensor/SensorIn.ASensor
  T_out_c : Outport
  wires:
  T_in_c/1 -> Discrete Derivative/1, Sum/2
  >8/1 -> Multiply/2  "W/m^2K"
  m*c/A/1 -> Multiply/1
  v_m/s/1 -> Compare To Constant/1, 1-D Lookup Table/1
  1-D Lookup Table/1 -> >8/1
  Multiply/1 -> Sum/1  "K"
  Multiply1/1 -> PT1 1sec1/1
  Discrete Derivative/1 -> Multiply1/3, -10<x<10 K/s/1
  PT1 1sec1/1 -> Multiply/3
  Compare To Constant/1 -> Data Type Conversion/1
  Data Type Conversion/1 -> Multiply1/1
  -10<x<10 K/s/1 -> Data Type Conversion1/1
  Data Type Conversion1/1 -> Multiply1/2
  Sum/1 -> -30<TGas<900degC/1
  -30<TGas<900degC/1 -> T_out_c/1

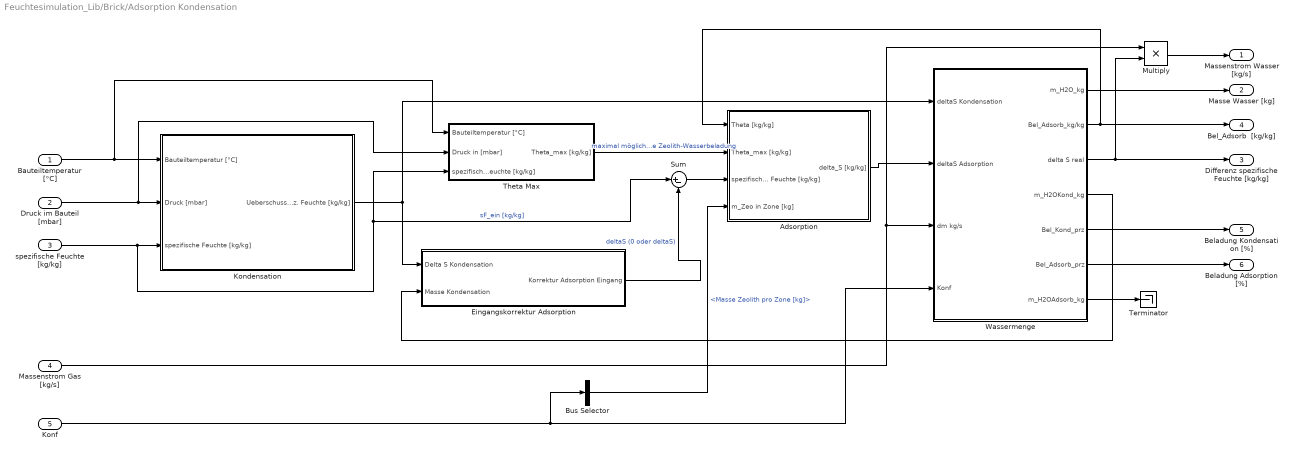
== system Feuchtesimulation_Lib/Brick/Adsorption Kondensation ==
  Bauteiltemperatur [°C] : Inport
  Druck im Bauteil [mbar] : Inport  Port=2
  spezifische Feuchte [kg/kg] : Inport  Port=3
  Massenstrom Gas [kg/s] : Inport  Port=4
  Konf : Inport  Port=5
  "Adsorption " : Subsystem
  Bus Selector : BusSelector  OutputSignals=Masse Zeolith pro Zone [kg]
  Eingangskorrektur Adsorption : Subsystem
  Kondensation : Subsystem
  Multiply : Product
  Sum : Sum  Inputs=|+-
  Terminator : Terminator
  "Theta Max " : Subsystem
  "Wassermenge " : Subsystem
  Massenstrom Wasser [kg/s] : Outport
  Masse Wasser [kg] : Outport  Port=2
  Differenz spezifische Feuchte [kg/kg] : Outport  Port=3
  Bel_Adsorb  [kg/kg] : Outport  Port=4
  Beladung Kondensation [%] : Outport  Port=5
  Beladung Adsorption [%] : Outport  Port=6
  wires:
  Kondensation/1(Ueberschuss spez. Feuchte [kg/kg]) -> Eingangskorrektur Adsorption/1(Delta S Kondensation), "Wassermenge "/1(deltaS Kondensation)
  spezifische Feuchte [kg/kg]/1 -> Sum/1, "Theta Max "/3(spezifische Feuchte [kg/kg]), Kondensation/3(spezifische Feuchte [kg/kg])  "sF_ein [kg/kg]"
  "Theta Max "/1(Theta_max [kg/kg]) -> "Adsorption "/2(Theta_max [kg/kg])  "maximal mögliche Zeolith-Wasserbeladung"
  Druck im Bauteil [mbar]/1 -> "Theta Max "/2(Druck in [mbar]), Kondensation/2(Druck [mbar])
  Konf/1 -> Bus Selector/1, "Wassermenge "/4(Konf)
  "Adsorption "/1(delta_S [kg/kg]) -> "Wassermenge "/2(deltaS Adsorption)
  Bauteiltemperatur [°C]/1 -> "Theta Max "/1(Bauteiltemperatur [°C]), Kondensation/1(Bauteiltemperatur [°C])
  Eingangskorrektur Adsorption/1(Korrektur Adsorption Eingang) -> Sum/2  "deltaS (0 oder deltaS)"
  Sum/1 -> "Adsorption "/3(spezifische Feuchte [kg/kg])
  Massenstrom Gas [kg/s]/1 -> Multiply/1, "Wassermenge "/3(dm kg/s)
  "Wassermenge "/4(m_H2OKond_kg) -> Eingangskorrektur Adsorption/2(Masse Kondensation)
  "Wassermenge "/1(m_H2O_kg) -> Masse Wasser [kg]/1
  "Wassermenge "/3(delta S real) -> Multiply/2, Differenz spezifische Feuchte [kg/kg]/1
  "Wassermenge "/5(Bel_Kond_prz) -> Beladung Kondensation [%]/1
  Multiply/1 -> Massenstrom Wasser [kg/s]/1
  "Wassermenge "/6(Bel_Adsorb_prz) -> Beladung Adsorption [%]/1
  "Wassermenge "/7(m_H2OAdsorb_kg) -> Terminator/1
  Bus Selector/1 -> "Adsorption "/4(m_Zeo in Zone [kg])  "<Masse Zeolith pro Zone [kg]>"
  "Wassermenge "/2(Bel_Adsorb_kg/kg) -> "Adsorption "/1(Theta [kg/kg]), Bel_Adsorb  [kg/kg]/1

== system Feuchtesimulation_Lib/Brick/Enthalpiestrom ausgehend  ==
  Temperatur Gas ausgehend [°C] : Inport
  Massenstrom Gas [kg/s] : Inport  Port=2
  spezifische Feuchte [kg/kg] : Inport  Port=3
  dH_out_Jps : Product  Inputs=***
  kombinierte Wärmekapazität : Subsystem
  Enthalpiestrom ausgehend [W] : Outport
  wires:
  dH_out_Jps/1 -> Enthalpiestrom ausgehend [W]/1
  spezifische Feuchte [kg/kg]/1 -> kombinierte Wärmekapazität/1(Spezifische Feuchte)
  kombinierte Wärmekapazität/1(kombinierte Wärmekapazität) -> dH_out_Jps/3
  Massenstrom Gas [kg/s]/1 -> dH_out_Jps/2
  Temperatur Gas ausgehend [°C]/1 -> dH_out_Jps/1

== system Feuchtesimulation_Lib/Brick/Enthalpiestrom eingehend  ==
  Temperatur Gas eingehend [°C] : Inport
  Massenstrom Gas [kg/s] : Inport  Port=2
  spezifische Feuchte [kg/kg] : Inport  Port=3
  Multiply : Product  Inputs=***
  kombinierte Wärmekapazität : Subsystem
  Enthalpiestrom eingehend [W] : Outport
  wires:
  Multiply/1 -> Enthalpiestrom eingehend [W]/1
  Massenstrom Gas [kg/s]/1 -> Multiply/2
  spezifische Feuchte [kg/kg]/1 -> kombinierte Wärmekapazität/1(Spezifische Feuchte)
  Temperatur Gas eingehend [°C]/1 -> Multiply/1
  kombinierte Wärmekapazität/1(kombinierte Wärmekapazität) -> Multiply/3

== system Feuchtesimulation_Lib/Brick/Trägheit  ==
  Temperatur Bauteil [°C] : Inport
  Masse Wasser [kg] : Inport  Port=2
  Konf : Inport  Port=3
  Bus Selector : BusSelector  OutputSignals=Material Bauteil.Wärmekapazität KL Temperatur [°C],Material Bauteil.Wärmekapazität Kennlienie [kJ/kgK],Masse Bauteil pro Zone [kg]
  Constant : Constant  Value=waermekapazitaet_wasser_fluessig
  Multiply : Product
  Sum : Sum  Inputs=++|
  Wärmekapazität : simulink/Lookup Tables/Lookup Table Dynamic  LookUpMeth=Interpolation-Use End Values  OutDataType=fixdt('single')  OutScaling=[]  OutputDataTypeScalingMode=Specify via dialog  OutDataTypeStr=fixdt('single')  RndMeth=Simplest  DoSatur=off
      settings: SourceProductName=Simulink
  kJ2J : Gain  Gain=1000
  mc : Product
  m*c_J/K : Outport
  wires:
  Bus Selector/3 -> mc/2  "<Masse Bauteil pro Zone [kg]>"
  kJ2J/1 -> mc/1
  Temperatur Bauteil [°C]/1 -> Wärmekapazität/1
  Konf/1 -> Bus Selector/1
  Bus Selector/1 -> Wärmekapazität/2  "<Wärmekapazität KL Temperatur [°C]>"
  Bus Selector/2 -> Wärmekapazität/3  "<Wärmekapazität Kennlienie [kJ/kgK]>"
  Wärmekapazität/1 -> kJ2J/1
  mc/1 -> Sum/2  "J/kg"
  Sum/1 -> m*c_J/K/1
  Masse Wasser [kg]/1 -> Multiply/2
  Constant/1 -> Multiply/1
  Multiply/1 -> Sum/1  "J/kg"

== system Feuchtesimulation_Lib/Brick/Wärmeleitung ausgehend  ==
  note: Q_WL = deltaT * (A * AeffFaktor) / (Lges / Nzonen) * lambda
  Temperatur Bauteil (=Ausgehend) [°C] : Inport
  Temperatur nächste Zone [°C] : Inport  Port=2
  Konf : Inport  Port=3
  Bus Selector : BusSelector  OutputSignals=Querschnittsfläche Bauteil [m2],Gesamtlänge Bauteil [m],Anzahl Zonen [-],Material Bauteil,Material Bauteil.AeffFaktor [-]
  Bus Selector1 : BusSelector  OutputSignals=Wärmeleitfähigkeit [W/mK]
  Divide : Product  Inputs=**/***
  Sum : Sum  Inputs=|+-
  Wärmestrom ausgehend [W] : Outport
  wires:
  Temperatur nächste Zone [°C]/1 -> Sum/2
  Temperatur Bauteil (=Ausgehend) [°C]/1 -> Sum/1
  Divide/1 -> Wärmestrom ausgehend [W]/1
  Sum/1 -> Divide/1
  Konf/1 -> Bus Selector/1
  Bus Selector/1 -> Divide/2  "<Querschnittsfläche Bauteil [m2]>"
  Bus Selector/2 -> Divide/3  "<Gesamtlänge Bauteil [m]>"
  Bus Selector/4 -> Bus Selector1/1  "<Material Bauteil>"
  Bus Selector1/1 -> Divide/5  "<Wärmeleitfähigkeit [W/mK]>"
  Bus Selector/3 -> Divide/4  "<Anzahl Zonen [-]>"
  Bus Selector/5 -> Divide/6  "<AeffFaktor [-]>"

== system Feuchtesimulation_Lib/Brick/Wärmeleitung eingehend ==
  note: Q_WL = deltaT * (A * AeffFaktor) / (Lges / Nzonen) * lambda
  Temperatur eingehen [°C] : Inport
  Temperatur ausgehend [°C] : Inport  Port=2
  Konf : Inport  Port=3
  Bus Selector : BusSelector  OutputSignals=Querschnittsfläche Bauteil [m2],Gesamtlänge Bauteil [m],Anzahl Zonen [-],Material Bauteil,Material Bauteil.AeffFaktor [-]
  Bus Selector1 : BusSelector  OutputSignals=Wärmeleitfähigkeit [W/mK]
  Divide : Product  Inputs=**/***
  Sum : Sum  Inputs=|+-
  Wärmestrom eingehen [W] : Outport
  wires:
  Temperatur ausgehend [°C]/1 -> Sum/2
  Temperatur eingehen [°C]/1 -> Sum/1
  Divide/1 -> Wärmestrom eingehen [W]/1
  Sum/1 -> Divide/1
  Bus Selector1/1 -> Divide/5  "<Wärmeleitfähigkeit [W/mK]>"
  Bus Selector/4 -> Bus Selector1/1  "<Material Bauteil>"
  Konf/1 -> Bus Selector/1
  Bus Selector/5 -> Divide/6  "<AeffFaktor [-]>"
  Bus Selector/1 -> Divide/2  "<Querschnittsfläche Bauteil [m2]>"
  Bus Selector/3 -> Divide/4  "<Anzahl Zonen [-]>"
  Bus Selector/2 -> Divide/3  "<Gesamtlänge Bauteil [m]>"

== system Feuchtesimulation_Lib/Brick/dQ Desorption\Verdunstung ==
  Massenstrom Wasser [kg/s] : Inport
  Theta (Beladung Adsorption) : Inport  Port=2
  Adsorptionsenthalpie : Lookup_n-D  NumberOfTableDimensions=1  BreakpointsForDimension1=adsorptionsenthalpie.x  Table=adsorptionsenthalpie.h  InternalRulePriority=Speed  RndMeth=Simplest  InputSameDT=on
  dQa : Product
  kJ to J : Gain  Gain=1e3
  Wärmestrom Adsorption/Kondensation [W] : Outport
  wires:
  Adsorptionsenthalpie/1 -> kJ to J/1
  Massenstrom Wasser [kg/s]/1 -> dQa/1
  dQa/1 -> Wärmestrom Adsorption/Kondensation [W]/1
  kJ to J/1 -> dQa/2
  Theta (Beladung Adsorption)/1 -> Adsorptionsenthalpie/1  "Theta"

== system Feuchtesimulation_Lib/Rohrwandabschnitt/Gastemperatur_im_Rohr_Integration ==
  note: H mit Basis degC!!!
  note: Kein Unit Delay nötig wegen discrete Integrator vermutlich
  Q_Gas-Wand [W] : Inport
  mpkt [kgps] : Inport  Port=2
  Hein [W] : Inport  Port=3
  Fspez_kg/kg : Inport  Port=4
  T_init_degC : Inport  Port=5
  Discrete-Time Integrator1 : DiscreteIntegrator  ExternalReset=rising  InitialConditionSource=external  SampleTime=-1  LimitOutput=on  UpperSaturationLimit=999  LowerSaturationLimit=-273  ICPrevOutput=DiscIntNeverNeededParam  ICPrevScaledInput=DiscIntNeverNeededParam
  Haus [W] : Product  Inputs=***
  Hein-Haus-QWand2Gas [W] : Sum  Inputs=--+
  SummeQ/m/cp : Product  Inputs=*//
  kombinierte Wärmekapazität : $bdroot/Brick/Enthalpiestrom eingehend /kombinierte Wärmekapazität  SystemSampleTime=-1
  mGas [kg] im Rohrabschnitt konstant : Constant  Value=mGas_imRohrabschnitt_kg
  T_Gas  °C : Outport
  H_aus_W : Outport  Port=2
  wires:
  Discrete-Time Integrator1/1 -> Haus [W]/1, T_Gas  °C/1  "TGas °C"
  T_init_degC/1 -> Discrete-Time Integrator1/3
  kombinierte Wärmekapazität/1 -> Haus [W]/2, SummeQ/m/cp/3  "J/kgK"
  SummeQ/m/cp/1 -> Discrete-Time Integrator1/1  "deltaT/deltat [K/s]"
  mpkt [kgps]/1 -> Haus [W]/3
  Hein [W]/1 -> Hein-Haus-QWand2Gas [W]/3
  Haus [W]/1 -> H_aus_W/1, Hein-Haus-QWand2Gas [W]/2
  Q_Gas-Wand [W]/1 -> Hein-Haus-QWand2Gas [W]/1
  Hein-Haus-QWand2Gas [W]/1 -> SummeQ/m/cp/1
  mGas [kg] im Rohrabschnitt konstant/1 -> SummeQ/m/cp/2
  Fspez_kg/kg/1 -> kombinierte Wärmekapazität/1
  [TempInit_ResetSignal_0oder1] -> Discrete-Time Integrator1/2

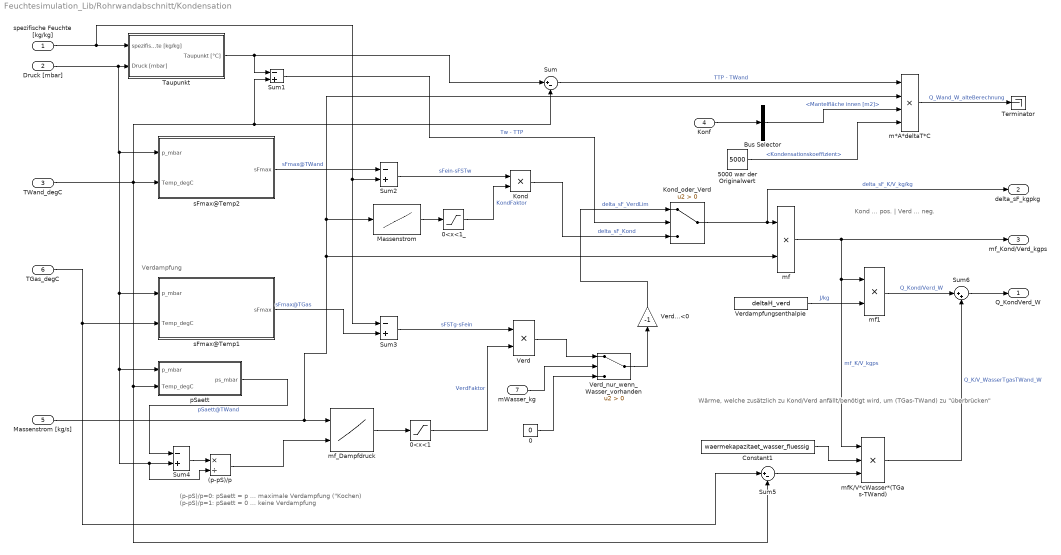
== system Feuchtesimulation_Lib/Rohrwandabschnitt/Kondensation ==
  note: Kond ... pos. | Verd ... neg.
  note: Wärme, welche zusätzlich zu Kond/Verd anfällt/benötigt wird,
      | um (TGas-TWand) zu "überbrücken"
  note: Verdampfung
  note: (p-pS)/p=0:   pSaett = p ... maximale Verdampfung ("Kochen)
      | (p-pS)/p=1:   pSaett = 0 ... keine Verdampfung
  spezifische Feuchte [kg/kg] : Inport
  Druck [mbar] : Inport  Port=2
  TWand_degC : Inport  Port=3
  Konf : Inport  Port=4
  Massenstrom [kg/s] : Inport  Port=5
  TGas_degC : Inport  Port=6
  mWasser_kg : Inport  Port=7
  (p-pS)/p : Product  Inputs=*/
  0 : Constant  Value=0
  0<x<1 : Saturate  UpperLimit=1  LowerLimit=0
  0<x<1_ : Saturate  UpperLimit=1  LowerLimit=0
  5000 war der Originalwert : Constant  Value=5000
  Bus Selector : BusSelector  OutputSignals=Mantelfläche innen [m2]
  Constant1 : Constant  Value=waermekapazitaet_wasser_fluessig
  Kond : Product
  Kond_oder_Verd : Switch  Criteria=u2 > Threshold
  Massenstrom : Lookup_n-D  NumberOfTableDimensions=1  BreakpointsForDimension1=KondVerd_KLKF_mf_StSt_kgps  Table=Kond_KL_Faktor_  InternalRulePriority=Speed  RndMeth=Simplest  InputSameDT=on
  Sum : Sum  Inputs=|+-
  Sum{1..4} (4 alike) : Sum  Inputs=-+
  Sum5 : Sum  Inputs=|+-
  Sum6 : Sum  Inputs=|++
  Taupunkt : Subsystem
  Terminator : Terminator
  Verd : Product
  Verd...<0 : Gain  Gain=-1
  Verd_nur_wenn_Wasser_vorhanden : Switch  Criteria=u2 > Threshold
  Verdampfungsenthalpie : Constant  Value=deltaH_verd
  m*A*deltaT*C : Product  Inputs=4
  mf : Product
  mf1 : Product
  mfK/V*cWasser*(TGas-TWand) : Product  Inputs=***
  mf_Dampfdruck : Lookup_n-D  BreakpointsForDimension1=KondVerd_KLKF_mf_StSt_kgps  BreakpointsForDimension2=Verd_KF_Dampfdruck_StSt  Table=Verd_KL_Faktor  ExtrapMethod=Clip  InternalRulePriority=Speed  RndMeth=Simplest  InputSameDT=on
  pSaett : MATLAB Function  TreatAsAtomicUnit=on
  sFmax@Temp1 : MATLAB Function  TreatAsAtomicUnit=on
  sFmax@Temp2 : MATLAB Function  TreatAsAtomicUnit=on
  Q_KondVerd_W : Outport
  delta_sF_kgpkg : Outport  Port=2
  mf_Kond/Verd_kgps : Outport  Port=3
  wires:
  spezifische Feuchte [kg/kg]/1 -> Sum3/1, Sum2/2, Taupunkt/1(spezifische Feuchte [kg/kg])
  Taupunkt/1(Taupunkt [°C]) -> Sum1/1, Sum/1
  5000 war der Originalwert/1 -> m*A*deltaT*C/4  "<Kondensationskoeffizient>"
  Konf/1 -> Bus Selector/1
  Sum/1 -> m*A*deltaT*C/1  "TTP - TWand"
  Bus Selector/1 -> m*A*deltaT*C/3  "<Mantelfläche innen [m2]>"
  sFmax@Temp2/1(sFmax) -> Sum2/1  "sFmax@TWand"
  sFmax@Temp1/1(sFmax) -> Sum3/2  "sFmax@TGas"
  mf_Dampfdruck/1 -> 0<x<1/1
  Massenstrom [kg/s]/1 -> Massenstrom/1, m*A*deltaT*C/2, mf/2, mf_Dampfdruck/1
  0<x<1/1 -> Verd/2  "VerdFaktor"
  Sum1/1 -> Kond_oder_Verd/2  "Tw - TTP"
  Sum2/1 -> Kond/1  "sFein-sFSTw"
  Sum3/1 -> Verd/1  "sFSTg-sFein"
  Kond/1 -> Kond_oder_Verd/3  "delta_sF_Kond"
  Kond_oder_Verd/1 -> delta_sF_kgpkg/1, mf/1  "delta_sF_K/V_kg/kg"
  Verdampfungsenthalpie/1 -> mf1/2  "J/kg"
  mf/1 -> mfK/V*cWasser*(TGas-TWand)/1, mf1/1, mf_Kond/Verd_kgps/1  "mf_K/V_kgps"
  mWasser_kg/1 -> Verd_nur_wenn_Wasser_vorhanden/2
  Verd_nur_wenn_Wasser_vorhanden/1 -> Verd...<0/1
  Verd/1 -> Verd_nur_wenn_Wasser_vorhanden/1
  0/1 -> Verd_nur_wenn_Wasser_vorhanden/3
  Verd...<0/1 -> Kond_oder_Verd/1  "delta_sF_VerdLim"
  Druck [mbar]/1 -> sFmax@Temp2/1(p_mbar), (p-pS)/p/2, Sum4/2, pSaett/1(p_mbar), sFmax@Temp1/1(p_mbar), Taupunkt/2(Druck [mbar])
  pSaett/1(ps_mbar) -> Sum4/1  "pSaett@TWand"
  Sum4/1 -> (p-pS)/p/1
  (p-pS)/p/1 -> mf_Dampfdruck/2
  Massenstrom/1 -> 0<x<1_/1
  TGas_degC/1 -> Sum5/1, sFmax@Temp1/2(Temp_degC)
  TWand_degC/1 -> Sum5/2, pSaett/2(Temp_degC), sFmax@Temp2/2(Temp_degC), Sum1/2, Sum/2
  Sum5/1 -> mfK/V*cWasser*(TGas-TWand)/3
  Constant1/1 -> mfK/V*cWasser*(TGas-TWand)/2
  mfK/V*cWasser*(TGas-TWand)/1 -> Sum6/2  "Q_K/V_WasserTgasTWand_W"
  mf1/1 -> Sum6/1  "Q_Kond/Verd_W"
  Sum6/1 -> Q_KondVerd_W/1
  m*A*deltaT*C/1 -> Terminator/1  "Q_Wand_W_alteBerechnung"
  0<x<1_/1 -> Kond/2  "KondFaktor"

== system Feuchtesimulation_Lib/Rohrwandabschnitt/Q Gas an Wand ==
  Wandtemperatur[°C] : Inport
  T_Gas_degC : Inport  Port=2
  Druck [mbar] : Inport  Port=3
  Massenstrom [kg/s] : Inport  Port=4
  Konf : Inport  Port=5
  Alpha Gas Wand : $bdroot/Alpha Gas Wand  SystemSampleTime=-1
  Bus Selector : BusSelector  OutputSignals=Mantelfläche innen [m2],gleichwertiger Strömungsdurchmesser [m]
  Korr. für erhöhten Wü wegen instationärer Strömung : Gain  Gain=WuezRohr_Dynamikfaktor
  Sum : Sum  Inputs=|-+
  alfa*deltaT*A : Product  Inputs=3
  dm_2_v : Subsystem
  Q_Gas_zu_Wand [W] : Outport
  wires:
  Bus Selector/1 -> alfa*deltaT*A/3  "<Mantelfläche innen [m2]>"
  Druck [mbar]/1 -> dm_2_v/2(p_mbar)
  Sum/1 -> alfa*deltaT*A/1  "TGas - TWand"
  Wandtemperatur[°C]/1 -> Sum/1
  dm_2_v/1(v_m/s) -> Alpha Gas Wand/2
  Bus Selector/2 -> dm_2_v/4(D_eff_m), Alpha Gas Wand/3  "<gleichwertiger Strömungsdurchmesser [m]>"
  Massenstrom [kg/s]/1 -> dm_2_v/1(dm_kg/s)
  Konf/1 -> Bus Selector/1
  T_Gas_degC/1 -> Alpha Gas Wand/1, Sum/2, dm_2_v/3(Tg_C)
  alfa*deltaT*A/1 -> Q_Gas_zu_Wand [W]/1
  Alpha Gas Wand/1 -> Korr. für erhöhten Wü wegen instationärer Strömung/1  "alfa"
  Korr. für erhöhten Wü wegen instationärer Strömung/1 -> alfa*deltaT*A/2

== system Feuchtesimulation_Lib/Rohrwandabschnitt/Q Wand an Umg ==
  note: WÜZ innen Gas-->Rohr wird ignoriert
  note: Q_aussen = A * 1/r_ges * delta_T
  note: Alfa für Quer-Umströmung eines Zylinders mit 150mm Durchm.
      | @ 0 bis 20°C, 1bar
  Wandtemperatur [°C] : Inport
  Umgebungstemperatur [°C] : Inport  Port=2
  Konf : Inport  Port=3
  1-D Lookup Table : Lookup_n-D  NumberOfTableDimensions=1  BreakpointsForDimension1=[0, 10, 20, 50, 100, 200, 300]  Table=[8, 18, 32, 66, 116, 200, 280]  InternalRulePriority=Speed  RndMeth=Simplest  InputSameDT=on
  Bus Selector : BusSelector  OutputSignals=r_thermWidIso_m2K/W,r_thermWidRohr_m2K/W,Mantelfläche außen [m2]
  Constant : Constant
  From Workspace : FromWorkspace  VariableName=VehV_v  SampleTime=0
  Multiply : Product  Inputs=/**
  Multiply1 : Product  Inputs=*/
  Sum : Sum  Inputs=|+-
  Sum1 : Sum  Inputs=+++
  Wärmestrom [W] : Outport
  wires:
  Wandtemperatur [°C]/1 -> Sum/1
  Umgebungstemperatur [°C]/1 -> Sum/2
  Sum/1 -> Multiply/2
  Multiply/1 -> Wärmestrom [W]/1
  Konf/1 -> Bus Selector/1
  Bus Selector/3 -> Multiply/3  "<Mantelfläche außen [m2]>"
  From Workspace/1 -> 1-D Lookup Table/1
  1-D Lookup Table/1 -> Multiply1/2  "alfa_aussen_W/m2K"
  Bus Selector/1 -> Sum1/2  "<r_thermWidIso_m2K/W>"
  Bus Selector/2 -> Sum1/3  "<r_thermWidRohr_m2K/W>"
  Constant/1 -> Multiply1/1
  Multiply1/1 -> Sum1/1
  Sum1/1 -> Multiply/1  "r_ges_m2K/W"

== system Feuchtesimulation_Lib/Rohrwandabschnitt/Trägheit Rohr ==
  Konf : Inport
  Bus Selector : BusSelector  OutputSignals=Wärmekapazität Rohr [J/kgK],Masse Rohr [kg]
  Multiply : Product
  m*c : Outport
  wires:
  Konf/1 -> Bus Selector/1
  Bus Selector/1 -> Multiply/1  "<Wärmekapazität Rohr [J/kgK]>"
  Bus Selector/2 -> Multiply/2  "<Masse Rohr [kg]>"
  Multiply/1 -> m*c/1

== system Feuchtesimulation_Lib/Rohrwandabschnitt/Wärmeleitung Downstream ==
  note: Q_WL_vorherigesRohr = A * delta_T * lambda / L
  Wandtemperatur[°C] : Inport
  Temperatur nächster Abschnitt [°C] : Inport  Port=2
  Konf : Inport  Port=3
  Bus Selector : BusSelector  OutputSignals=Wärmeleitfähigkeit [W/mK],Länge RohrSegment [m],Wärmeleitquerschnitt Rohr [m2]
  Divide : Product  Inputs=**/*
  Sum : Sum  Inputs=|+-
  Wärmestrom_nach_Ds [W] : Outport
  wires:
  Konf/1 -> Bus Selector/1
  Sum/1 -> Divide/1
  Divide/1 -> Wärmestrom_nach_Ds [W]/1
  Wandtemperatur[°C]/1 -> Sum/1
  Temperatur nächster Abschnitt [°C]/1 -> Sum/2
  Bus Selector/1 -> Divide/2  "<Wärmeleitfähigkeit [W/mK]>"
  Bus Selector/3 -> Divide/4  "<Wärmeleitquerschnitt Rohr [m2]>"
  Bus Selector/2 -> Divide/3  "<Länge RohrSegment [m]>"

== system Feuchtesimulation_Lib/Rohrwandabschnitt/Wärmeleitung Upstream ==
  note: Q_WL_vorherigesRohr = A * delta_T * lambda / L
  Temperatur vorheriger Abschnitt [°C] : Inport
  Wandtemperatur[°C] : Inport  Port=2
  Konf : Inport  Port=3
  Bus Selector : BusSelector  OutputSignals=Wärmeleitfähigkeit [W/mK],Länge RohrSegment [m],Wärmeleitquerschnitt Rohr [m2]
  Divide : Product  Inputs=**/*
  Sum : Sum  Inputs=|+-
  Wärmestrom_von_Us [W] : Outport
  wires:
  Konf/1 -> Bus Selector/1
  Sum/1 -> Divide/1  "T_Us - TWand"
  Divide/1 -> Wärmestrom_von_Us [W]/1
  Temperatur vorheriger Abschnitt [°C]/1 -> Sum/1
  Wandtemperatur[°C]/1 -> Sum/2
  Bus Selector/1 -> Divide/2  "<Wärmeleitfähigkeit [W/mK]>"
  Bus Selector/3 -> Divide/4  "<Wärmeleitquerschnitt Rohr [m2]>"
  Bus Selector/2 -> Divide/3  "<Länge RohrSegment [m]>"

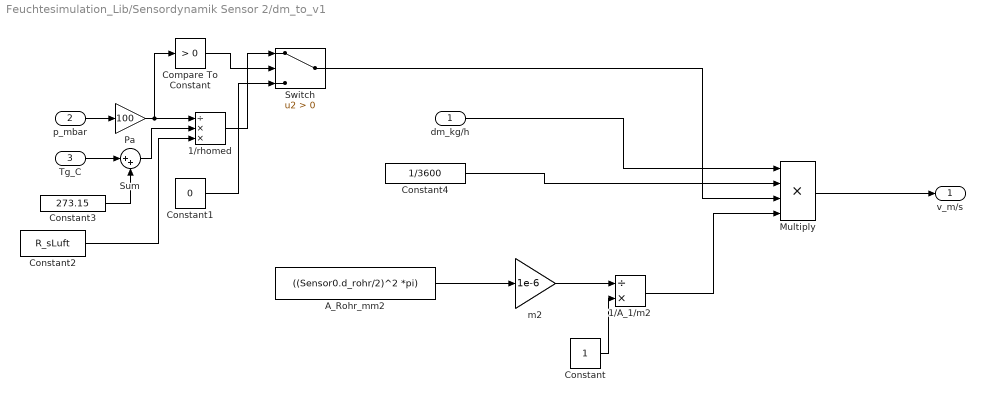
== system Feuchtesimulation_Lib/Sensordynamik Sensor 2/dm_to_v1 ==
  dm_kg/h : Inport
  p_mbar : Inport  Port=2
  Tg_C : Inport  Port=3
  1/A_1/m2 : Product  Inputs=/*
  1/rhomed : Product  Inputs=/**
  A_Rohr_mm2 : Constant  Value=((Sensor0.d_rohr/2)^2 *pi)
  Compare To Constant : simulink/Logic and Bit Operations/Compare To Constant  relop=>  const=0  OutDataTypeStr=boolean
  Constant : Constant
  Constant1 : Constant  Value=0
  Constant2 : Constant  Value=R_sLuft
  Constant3 : Constant  Value=273.15
  Constant4 : Constant  Value=1/3600
  Multiply : Product  Inputs=4
  Pa : Gain  Gain=100
  Sum : Sum  Inputs=|++
  Switch : Switch  Criteria=u2 > Threshold
  m2 : Gain  Gain=1e-6
  v_m/s : Outport
  wires:
  dm_kg/h/1 -> Multiply/1
  Constant4/1 -> Multiply/2
  A_Rohr_mm2/1 -> m2/1
  m2/1 -> 1/A_1/m2/1
  Constant/1 -> 1/A_1/m2/2
  1/A_1/m2/1 -> Multiply/4
  Multiply/1 -> v_m/s/1
  Constant2/1 -> 1/rhomed/3
  Sum/1 -> 1/rhomed/2
  Tg_C/1 -> Sum/1
  Constant3/1 -> Sum/2
  p_mbar/1 -> Pa/1
  Pa/1 -> Compare To Constant/1, 1/rhomed/1
  Constant1/1 -> Switch/3
  Compare To Constant/1 -> Switch/2
  1/rhomed/1 -> Switch/1
  Switch/1 -> Multiply/3

== system Feuchtesimulation_Lib/rate/s to e ==
  s : Inport
  p : Inport  Port=2
  Constant : Constant  Value=H2O_mw/AIR_mw
  Divide : Product  Inputs=*/
  Multiply : Product
  Multiply1 : Product
  Sum : Sum  Inputs=|-++
  e : Outport
  wires:
  p/1 -> Multiply/2
  Multiply1/1 -> Sum/1
  Constant/1 -> Sum/2, Multiply1/2
  s/1 -> Sum/3, Multiply1/1, Multiply/1
  Sum/1 -> Divide/2
  Multiply/1 -> Divide/1
  Divide/1 -> e/1

== system Feuchtesimulation_Lib/Brick/Adsorption Kondensation/Adsorption  ==
  note: Die Beladung nähert sich dem Gleichgewichtszustand
      | Theta = Thetamax an
  Theta [kg/kg] : Inport
  Theta_max [kg/kg] : Inport  Port=2
  spezifische Feuchte [kg/kg] : Inport  Port=3
  m_Zeo in Zone [kg] : Inport  Port=4
  >1e-4 : Saturate  UpperLimit=1  LowerLimit=1e-4
  Constant : Constant
  Constant1 : Constant  Value=0
  Divide : Product  Inputs=*/
  Gain : Gain  Gain=Ads_AusnutzungsFaktor
  Multiply : Product
  Sum : Sum  Inputs=+-|
  Switch : Switch  Criteria=u2 > Threshold  Threshold=mZeo_UnterDerZeo0angenommenWird
  delta_S [kg/kg] : Outport
  wires:
  spezifische Feuchte [kg/kg]/1 -> Gain/1
  Constant/1 -> Sum/1
  Divide/1 -> Sum/2
  Theta [kg/kg]/1 -> Divide/1
  Theta_max [kg/kg]/1 -> >1e-4/1
  >1e-4/1 -> Divide/2
  m_Zeo in Zone [kg]/1 -> Switch/2
  Multiply/1 -> Switch/1
  Constant1/1 -> Switch/3
  Switch/1 -> delta_S [kg/kg]/1
  Sum/1 -> Multiply/1
  Gain/1 -> Multiply/2
